simulink model "quadCorke"  (R2018a)
settings: Solver=VariableStepAuto  StartTime=0.0  StopTime=10.0  RelTol=1e-3
values from neighbouring files (symbols this model uses):
  MapMatrix = diag([ 1, -1, -1, -1, -1, 1, 1, -1, -1, -1, -1, 1])    [ScriptValues.m]
  x_d = 0    [ScriptValues.m]
  y_d = 0    [ScriptValues.m]
  z_d = 1    [ScriptValues.m]
undefined symbols (not defined in the file or in its folder): quadrotor
libraries: simulink x6, roblocks x2, aerolibutil x1
settings Model: Creator=dinies33  LastModifiedBy=giuseppe
settings ConfigComp: CovScope=ReferencedModels  CovIncludeTopModel=off

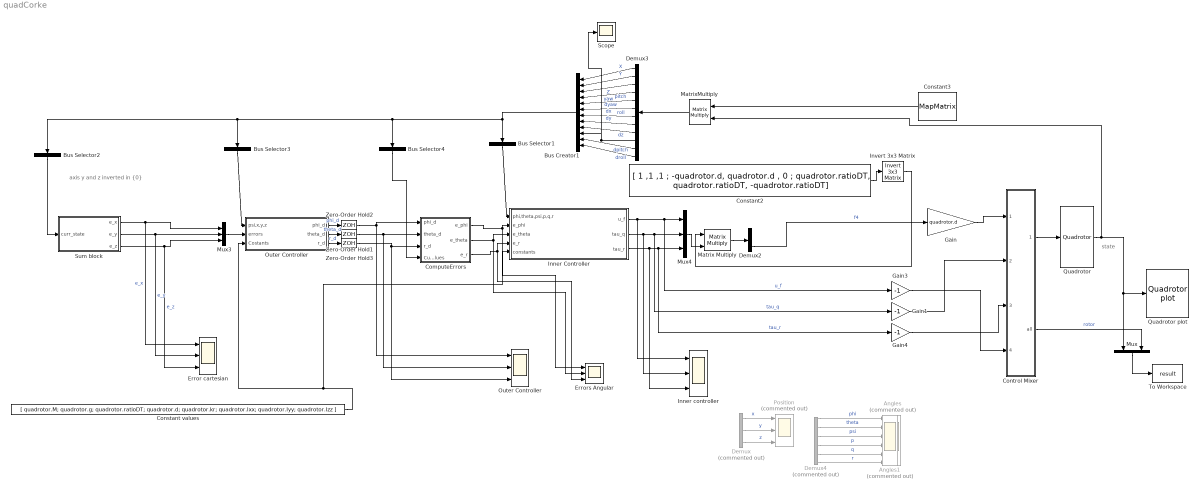
== system quadCorke ==
  note: axis y and z inverted in {0}
  note: state
  Angles : Scope  Commented=on  NumInputPorts=6
  Angles1 : Scope  Commented=on  NumInputPorts=6
  Bus Creator1 : BusCreator  Inputs='X','Y','Z','yaw','pitch','roll','dx','dy','dz','dyaw','dpitch','droll'
  Bus Selector1 : BusSelector  OutputSignals=roll,pitch,yaw,droll,dpitch,dyaw  OutputAsBus=on
  Bus Selector2 : BusSelector  OutputSignals=X,Y,Z  OutputAsBus=on
  Bus Selector3 : BusSelector  OutputSignals=yaw,X,Y,Z  OutputAsBus=on
  Bus Selector4 : BusSelector  OutputSignals=roll,pitch,dyaw  OutputAsBus=on
  "ComputeErrors " : Subsystem
  Constant values : Constant  Value=[ quadrotor.M; quadrotor.g; quadrotor.ratioDT; quadrotor.d; quadrotor.kr; quadrotor.Ixx; quadrotor.Iyy; quadrotor.Izz ]
  Constant2 : Constant  Value=[ 1 ,1 ,1 ; -quadrotor.d, quadrotor.d , 0 ; quadrotor.ratioDT, quadrotor.ratioDT, -quadrotor.ratioDT]
  Constant3 : Constant  Value=MapMatrix
  Control Mixer : Subsystem  AncestorBlock=roblocks/Vehicles/Control Mixer 4  mask{quad=quadrotor, maxrot=1000, minrot=5}
      mask prompts: quad "Quadrotor parameters"; maxrot "Maximum rotor speed (rad/s)"; minrot "Minimum rotor speed (rad/s)"
      mask help: Quadrotor control mixer
      mask Help:
      | Determine rotor speeds based on desired torques and thrust, and propellor model
      | 
      | <b>Inputs::</b>
      | tau<sub>x</sub> (1x1)    desired rolling torque [Nm]
      | 
      | tau<sub>y</sub> (1x1)    desired pitching torque [Nm]
      | tau<sub>z</sub> (1x1)    desired yawing torque [Nm]
      | T (1x1)          desired thrust [N]
      | 
      | <b>Outputs::</b>
      | 
      | w1 (1x1) angular velocity of rotor 1 [rad]
      | w2 (1x1) angular velocity of rotor 2 [rad]
      | w3 (1x1) angular velocity of rotor 3 [rad]
      | w4 (1x1) angular velocity of rotor 4 [rad]
      | 
      | <b>Notes::</b>
      | 
      | - Assumes the rotor labelling convention of RVC Fig 4.16.
      | - The quadrotor is underactuated and has only 4 inputs.
      mask Display:
      | port_label('output',1,'\varpi','texmode','on');
      | port_label('output',2,'\tau_a','texmode','on');
      | port_label('input',1,'\tau_x','texmode','on');
      | port_label('input',2,'\tau_y','texmode','on');
      | port_label('input',3,'\tau_z','texmode','on');
      | port_label('input',4,'T','texmode','on');
  Demux : Demux  Commented=on  Outputs=3
  Demux2 : Demux  Outputs=3
  Demux3 : Demux  Outputs=12
  Demux4 : Demux  Commented=on  Outputs=6
  Error cartesian : Scope  NumInputPorts=3
  Errors Angular : Scope  NumInputPorts=3
  Gain : Gain  Gain=quadrotor.d
  Gain1 : Gain  Gain=-1
  Gain3 : Gain  Gain=-1
  Gain4 : Gain  Gain=-1
  "Inner Controller " : Subsystem
  Inner controller : Scope  NumInputPorts=3
  Invert 3x3 Matrix : aerolibutil/Invert  3x3 Matrix
  Matrix Multiply : Product  Multiplication=Matrix(*)
  MatrixMultiply : Product  Multiplication=Matrix(*)
  Mux : Mux  Inputs=2
  Mux3 : Mux  Inputs=3
  Mux4 : Mux  Inputs=3
  Outer Controller : Scope  NumInputPorts=3
  "Outer Controller " : Subsystem
  Position : Scope  Commented=on  NumInputPorts=3
  Quadrotor : roblocks/Vehicles/Quadrotor  quad=quadrotor  x0=[0 0 -5]  groundflag=on
      link override Dynamics: FunctionName=corke_dynamics
  Quadrotor plot : roblocks/Vehicles/Quadrotor plot  quad=quadrotor  xydim=2  zdim=10
      link override Plotter: FunctionName=corke_plot  Parameters=[xydim, zdim], 1, 1,quad
  Scope : Scope
  Sum block : Subsystem
  To Workspace : ToWorkspace  VariableName=result  SampleTime=-1
  Zero-Order Hold1 : ZeroOrderHold  SampleTime=0.15
  Zero-Order Hold2 : ZeroOrderHold  SampleTime=0.15
  Zero-Order Hold3 : ZeroOrderHold  SampleTime=0.15
  wires:
  Control Mixer/2(all) -> Mux/2  "rotor"
  Mux/1 -> To Workspace/1
  Quadrotor/1 -> Quadrotor plot/1, Mux/1, MatrixMultiply/2
  Control Mixer/1(omega) -> Quadrotor/1
  Constant2/1 -> Invert 3x3 Matrix/1
  "Inner Controller "/1(u_f) -> Gain3/1, Mux4/1, Inner controller/1  "u_f"
  Demux4/6 -> Angles/6  "r"
  Demux4/1 -> Angles/1  "phi"
  Demux2/3 -> Gain/1  "f4"
  Sum block/1("e_x ") -> Error cartesian/1, Mux3/1  "e_x"
  Demux/2 -> Position/2  "y"
  Demux4/5 -> Angles/5  "q"
  "ComputeErrors "/1("e_phi ") -> Errors Angular/1, "Inner Controller "/2(e_phi)
  "ComputeErrors "/2(e_theta) -> Errors Angular/2, "Inner Controller "/3(e_theta)
  Matrix Multiply/1 -> Demux2/1
  Demux/1 -> Position/1  "x"
  "Inner Controller "/2(tau_q) -> Inner controller/2, Mux4/2, Gain1/1  "tau_q"
  Invert 3x3 Matrix/1 -> Matrix Multiply/1
  "Inner Controller "/3(tau_r) -> Inner controller/3, Gain4/1, Mux4/3  "tau_r"
  "Outer Controller "/3(r_d) -> Zero-Order Hold3/1  "r_d"
  "Outer Controller "/1("phi_d ") -> Zero-Order Hold2/1  "phi_d"
  "ComputeErrors "/3(e_r) -> Errors Angular/3, "Inner Controller "/4(e_r)
  Demux/3 -> Position/3  "z"
  Demux4/4 -> Angles/4  "p"
  Mux4/1 -> Matrix Multiply/2
  Demux4/3 -> Angles/3  "psi"
  Constant values/1 -> "Outer Controller "/3(Costants), "Inner Controller "/5(constants)
  Demux4/2 -> Angles/2  "theta"
  "Outer Controller "/2(theta_d) -> Zero-Order Hold1/1  "theta_d"
  Mux3/1 -> "Outer Controller "/2(errors)
  Sum block/2(e_y) -> Error cartesian/2, Mux3/2  "e_y"
  Sum block/3(e_z) -> Error cartesian/3, Mux3/3  "e_z"
  Gain/1 -> Control Mixer/1(tau roll)
  Bus Selector1/1 -> "Inner Controller "/1(phi,theta,psi,p,q,r)
  Bus Selector3/1 -> "Outer Controller "/1(psi,x,y,z)
  Bus Selector2/1 -> Sum block/1(curr_state)
  Bus Selector4/1 -> "ComputeErrors "/4(Curr_values)
  Constant3/1 -> MatrixMultiply/1
  Bus Creator1/1 -> Bus Selector2/1, Bus Selector3/1, Bus Selector4/1, Bus Selector1/1
  Demux3/3 -> Bus Creator1/3  "Z"
  Demux3/8 -> Bus Creator1/8  "dy"
  Demux3/7 -> Bus Creator1/7  "dx"
  Demux3/10 -> Scope/1, Bus Creator1/10  "dyaw"
  Demux3/5 -> Bus Creator1/5  "pitch"
  Demux3/2 -> Bus Creator1/2  "Y"
  Demux3/4 -> Bus Creator1/4  "yaw"
  Demux3/1 -> Bus Creator1/1  "X"
  Demux3/9 -> Bus Creator1/9  "dz"
  Demux3/11 -> Bus Creator1/11  "dpitch"
  Demux3/6 -> Bus Creator1/6  "roll"
  Demux3/12 -> Bus Creator1/12  "droll"
  MatrixMultiply/1 -> Demux3/1
  Gain1/1 -> Control Mixer/2(tau pitch)
  Gain3/1 -> Control Mixer/4(total thrust)
  Gain4/1 -> Control Mixer/3(tau yaw)
  Zero-Order Hold3/1 -> Outer Controller/3, "ComputeErrors "/3(r_d)
  Zero-Order Hold1/1 -> Outer Controller/2, "ComputeErrors "/2(theta_d)
  Zero-Order Hold2/1 -> "ComputeErrors "/1(phi_d), Outer Controller/1

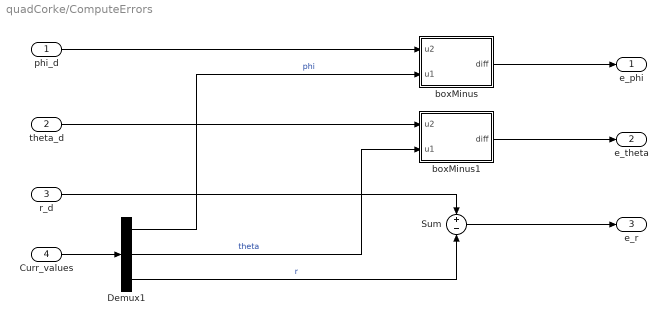
== system quadCorke/ComputeErrors  ==
  phi_d : Inport
  theta_d : Inport  Port=2
  r_d : Inport  Port=3
  Curr_values : Inport  Port=4
  Demux1 : Demux  Outputs=3
  Sum : Sum  Inputs=+-
  boxMinus : MATLAB Function  TreatAsAtomicUnit=on
  boxMinus1 : MATLAB Function  TreatAsAtomicUnit=on
  "e_phi " : Outport
  e_theta : Outport  Port=2
  e_r : Outport  Port=3
  wires:
  phi_d/1 -> boxMinus/1(u2)
  Demux1/1 -> boxMinus/2(u1)  "phi"
  theta_d/1 -> boxMinus1/1(u2)
  Demux1/2 -> boxMinus1/2(u1)  "theta"
  r_d/1 -> Sum/1
  Demux1/3 -> Sum/2  "r"
  Sum/1 -> e_r/1
  boxMinus1/1(diff) -> e_theta/1
  boxMinus/1(diff) -> "e_phi "/1
  Curr_values/1 -> Demux1/1

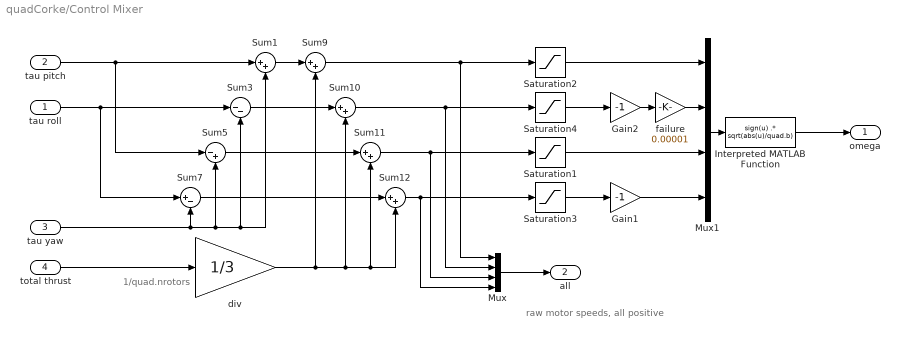
== system quadCorke/Control Mixer ==
  note: 1/quad.nrotors
  note: raw motor speeds, all positive
  tau roll : Inport
  tau pitch : Inport  Port=2
  tau yaw : Inport  Port=3
  total thrust : Inport  Port=4
  Gain1 : Gain  Gain=-1
  Gain2 : Gain  Gain=-1
  Interpreted MATLAB Function : MATLABFcn  MATLABFcn=sign(u) .* sqrt(abs(u)/quad.b)
  Mux : Mux
  Mux1 : Mux
  Saturation{1..4} (4 alike) : Saturate  UpperLimit=maxrot  LowerLimit=minrot
  Sum{1,9..12} (5 alike) : Sum  Inputs=|++  SaturateOnIntegerOverflow=on  InputSameDT=on  OutDataTypeStr=Inherit: Same as first input
  Sum3 : Sum  Inputs=|--  SaturateOnIntegerOverflow=on  InputSameDT=on  OutDataTypeStr=Inherit: Same as first input
  Sum5 : Sum  Inputs=|-+  SaturateOnIntegerOverflow=on  InputSameDT=on  OutDataTypeStr=Inherit: Same as first input
  Sum7 : Sum  Inputs=|+-  SaturateOnIntegerOverflow=on  InputSameDT=on  OutDataTypeStr=Inherit: Same as first input
  div : Gain  Gain=1/3
  failure : Gain  Gain=0.00001
  omega : Outport
  all : Outport  Port=2
  wires:
  div/1 -> Sum11/2, Sum12/2, Sum10/2, Sum9/2
  Interpreted MATLAB Function/1 -> omega/1
  Mux1/1 -> Interpreted MATLAB Function/1
  tau yaw/1 -> Sum7/2, Sum5/2, Sum3/2, Sum1/2
  Saturation2/1 -> Mux1/1
  Saturation4/1 -> Gain2/1
  Saturation1/1 -> Mux1/3
  Saturation3/1 -> Gain1/1
  tau pitch/1 -> Sum1/1, Sum5/1
  Sum1/1 -> Sum9/1
  Sum3/1 -> Sum10/1
  Sum5/1 -> Sum11/1
  Sum7/1 -> Sum12/1
  Sum9/1 -> Saturation2/1, Mux/1
  Sum10/1 -> Mux/2, Saturation4/1
  Sum11/1 -> Mux/3, Saturation1/1
  Sum12/1 -> Mux/4, Saturation3/1
  total thrust/1 -> div/1
  tau roll/1 -> Sum3/1, Sum7/1
  Mux/1 -> all/1
  Gain1/1 -> Mux1/4
  Gain2/1 -> failure/1
  failure/1 -> Mux1/2

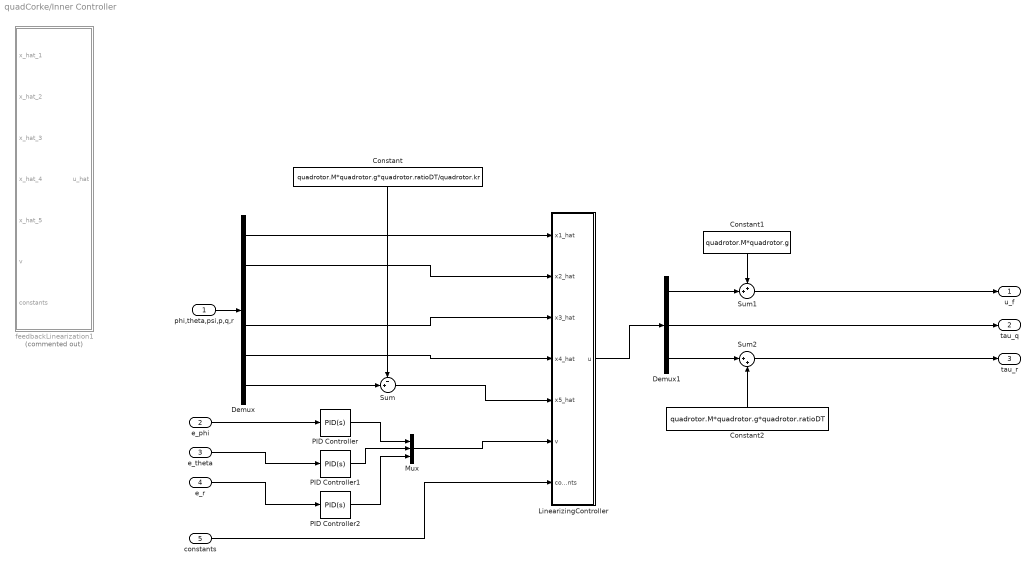
== system quadCorke/Inner Controller  ==
  phi,theta,psi,p,q,r : Inport
  e_phi : Inport  Port=2
  e_theta : Inport  Port=3
  e_r : Inport  Port=4
  constants : Inport  Port=5
  Constant : Constant  Value=quadrotor.M*quadrotor.g*quadrotor.ratioDT/quadrotor.kr
  Constant1 : Constant  Value=quadrotor.M*quadrotor.g
  Constant2 : Constant  Value=quadrotor.M*quadrotor.g*quadrotor.ratioDT
  Demux : Demux  Outputs=6
  Demux1 : Demux  Outputs=3
  LinearizingController : MATLAB Function  TreatAsAtomicUnit=on
  Mux : Mux  Inputs=3
  PID Controller : simulink/Continuous/PID Controller  Controller=PID  TimeDomain=Continuous-time  SampleTime=-1  IntegratorMethod=Forward Euler  FilterMethod=Forward Euler  Form=Parallel  UseFilter=on  ControllerParametersSource=internal  P=1  I=1  D=0  N=100  InitialConditionSource=internal  InitialConditionForIntegrator=0  InitialConditionForFilter=0  ExternalReset=none  LimitOutput=off  UpperSaturationLimit=inf  LowerSaturationLimit=-inf  LinearizeAsGain=on  AntiWindupMode=none  Kb=1  TrackingMode=off  Kt=1  PParamMin=[]  PParamMax=[]  IParamMin=[]  IParamMax=[]  DParamMin=[]  DParamMax=[]  NParamMin=[]  NParamMax=[]  KbParamMin=[]  KbParamMax=[]  KtParamMin=[]  KtParamMax=[]  POutMin=[]  POutMax=[]  IOutMin=[]  IOutMax=[]  DOutMin=[]  DOutMax=[]  NOutMin=[]  NOutMax=[]  KbOutMin=[]  KbOutMax=[]  KtOutMin=[]  KtOutMax=[]  IntegratorOutMin=[]  IntegratorOutMax=[]  FilterOutMin=[]  FilterOutMax=[]  SumOutMin=[]  SumOutMax=[]  SumI1OutMin=[]  SumI1OutMax=[]  SumI2OutMin=[]  SumI2OutMax=[]  SumI3OutMin=[]  SumI3OutMax=[]  SumDOutMin=[]  SumDOutMax=[]  SaturationOutMin=[]  SaturationOutMax=[]  IntegratorContinuousStateAttributes=''  IntegratorStateMustResolveToSignalObject=off  IntegratorRTWStateStorageClass=Auto  FilterContinuousStateAttributes=''  FilterStateMustResolveToSignalObject=off  FilterRTWStateStorageClass=Auto  DifferentiatorICPrevScaledInput=0  DifferentiatorOutMin=[]  DifferentiatorOutMax=[]  FilterDiffOutCoefMin=[]  FilterDiffOutCoefMax=[]  SumDenOutMin=[]  SumDenOutMax=[]  SumNumOutMin=[]  SumNumOutMax=[]  ReciprocalOutMin=[]  ReciprocalOutMax=[]  DivideOutMin=[]  DivideOutMax=[]  TunerSelectOption=Transfer Function Based (PID Tuner App)
  PID Controller1 : simulink/Continuous/PID Controller  Controller=PID  TimeDomain=Continuous-time  SampleTime=-1  IntegratorMethod=Forward Euler  FilterMethod=Forward Euler  Form=Parallel  UseFilter=on  ControllerParametersSource=internal  P=1  I=1  D=0  N=100  InitialConditionSource=internal  InitialConditionForIntegrator=0  InitialConditionForFilter=0  ExternalReset=none  LimitOutput=off  UpperSaturationLimit=inf  LowerSaturationLimit=-inf  LinearizeAsGain=on  AntiWindupMode=none  Kb=1  TrackingMode=off  Kt=1  PParamMin=[]  PParamMax=[]  IParamMin=[]  IParamMax=[]  DParamMin=[]  DParamMax=[]  NParamMin=[]  NParamMax=[]  KbParamMin=[]  KbParamMax=[]  KtParamMin=[]  KtParamMax=[]  POutMin=[]  POutMax=[]  IOutMin=[]  IOutMax=[]  DOutMin=[]  DOutMax=[]  NOutMin=[]  NOutMax=[]  KbOutMin=[]  KbOutMax=[]  KtOutMin=[]  KtOutMax=[]  IntegratorOutMin=[]  IntegratorOutMax=[]  FilterOutMin=[]  FilterOutMax=[]  SumOutMin=[]  SumOutMax=[]  SumI1OutMin=[]  SumI1OutMax=[]  SumI2OutMin=[]  SumI2OutMax=[]  SumI3OutMin=[]  SumI3OutMax=[]  SumDOutMin=[]  SumDOutMax=[]  SaturationOutMin=[]  SaturationOutMax=[]  IntegratorContinuousStateAttributes=''  IntegratorStateMustResolveToSignalObject=off  IntegratorRTWStateStorageClass=Auto  FilterContinuousStateAttributes=''  FilterStateMustResolveToSignalObject=off  FilterRTWStateStorageClass=Auto  DifferentiatorICPrevScaledInput=0  DifferentiatorOutMin=[]  DifferentiatorOutMax=[]  FilterDiffOutCoefMin=[]  FilterDiffOutCoefMax=[]  SumDenOutMin=[]  SumDenOutMax=[]  SumNumOutMin=[]  SumNumOutMax=[]  ReciprocalOutMin=[]  ReciprocalOutMax=[]  DivideOutMin=[]  DivideOutMax=[]  TunerSelectOption=Transfer Function Based (PID Tuner App)
  PID Controller2 : simulink/Continuous/PID Controller  Controller=PID  TimeDomain=Continuous-time  SampleTime=-1  IntegratorMethod=Forward Euler  FilterMethod=Forward Euler  Form=Parallel  UseFilter=on  ControllerParametersSource=internal  P=1  I=1  D=0  N=100  InitialConditionSource=internal  InitialConditionForIntegrator=0  InitialConditionForFilter=0  ExternalReset=none  LimitOutput=off  UpperSaturationLimit=inf  LowerSaturationLimit=-inf  LinearizeAsGain=on  AntiWindupMode=none  Kb=1  TrackingMode=off  Kt=1  PParamMin=[]  PParamMax=[]  IParamMin=[]  IParamMax=[]  DParamMin=[]  DParamMax=[]  NParamMin=[]  NParamMax=[]  KbParamMin=[]  KbParamMax=[]  KtParamMin=[]  KtParamMax=[]  POutMin=[]  POutMax=[]  IOutMin=[]  IOutMax=[]  DOutMin=[]  DOutMax=[]  NOutMin=[]  NOutMax=[]  KbOutMin=[]  KbOutMax=[]  KtOutMin=[]  KtOutMax=[]  IntegratorOutMin=[]  IntegratorOutMax=[]  FilterOutMin=[]  FilterOutMax=[]  SumOutMin=[]  SumOutMax=[]  SumI1OutMin=[]  SumI1OutMax=[]  SumI2OutMin=[]  SumI2OutMax=[]  SumI3OutMin=[]  SumI3OutMax=[]  SumDOutMin=[]  SumDOutMax=[]  SaturationOutMin=[]  SaturationOutMax=[]  IntegratorContinuousStateAttributes=''  IntegratorStateMustResolveToSignalObject=off  IntegratorRTWStateStorageClass=Auto  FilterContinuousStateAttributes=''  FilterStateMustResolveToSignalObject=off  FilterRTWStateStorageClass=Auto  DifferentiatorICPrevScaledInput=0  DifferentiatorOutMin=[]  DifferentiatorOutMax=[]  FilterDiffOutCoefMin=[]  FilterDiffOutCoefMax=[]  SumDenOutMin=[]  SumDenOutMax=[]  SumNumOutMin=[]  SumNumOutMax=[]  ReciprocalOutMin=[]  ReciprocalOutMax=[]  DivideOutMin=[]  DivideOutMax=[]  TunerSelectOption=Transfer Function Based (PID Tuner App)
  Sum : Sum  Inputs=-+|
  Sum1 : Sum  Inputs=++|
  Sum2 : Sum  Inputs=|++
  feedbackLinearization1 : MATLAB Function  Commented=on  TreatAsAtomicUnit=on
  u_f : Outport
  tau_q : Outport  Port=2
  tau_r : Outport  Port=3
  wires:
  phi,theta,psi,p,q,r/1 -> Demux/1
  Demux/1 -> LinearizingController/1(x1_hat)
  Demux/2 -> LinearizingController/2(x2_hat)
  Demux/4 -> LinearizingController/3(x3_hat)
  Demux/5 -> LinearizingController/4(x4_hat)
  Constant/1 -> Sum/1
  Sum/1 -> LinearizingController/5(x5_hat)
  Demux1/3 -> Sum2/1
  Demux1/1 -> Sum1/2
  Constant1/1 -> Sum1/1
  Sum1/1 -> u_f/1
  Demux1/2 -> tau_q/1
  Constant2/1 -> Sum2/2
  Sum2/1 -> tau_r/1
  constants/1 -> LinearizingController/7(constants)
  Demux/6 -> Sum/2
  e_theta/1 -> PID Controller1/1
  PID Controller2/1 -> Mux/3
  PID Controller/1 -> Mux/1
  Mux/1 -> LinearizingController/6(v)
  PID Controller1/1 -> Mux/2
  e_r/1 -> PID Controller2/1
  e_phi/1 -> PID Controller/1
  LinearizingController/1(u) -> Demux1/1

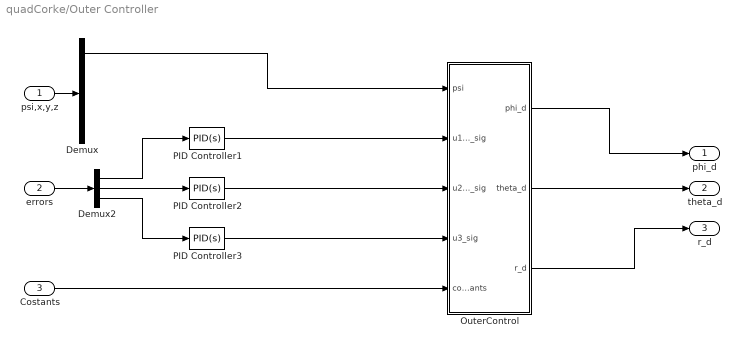
== system quadCorke/Outer Controller  ==
  psi,x,y,z : Inport  SampleTime=0.1
  errors : Inport  Port=2
  Costants : Inport  Port=3
  Demux : Demux
  Demux2 : Demux  Outputs=3
  OuterControl : MATLAB Function  TreatAsAtomicUnit=on
  PID Controller1 : simulink/Continuous/PID Controller  Controller=PID  TimeDomain=Continuous-time  SampleTime=-1  IntegratorMethod=Forward Euler  FilterMethod=Forward Euler  Form=Parallel  UseFilter=on  ControllerParametersSource=internal  P=0.939601981976548  I=0.0298455660718895  D=4.45438528962657  N=508.848592355901  InitialConditionSource=internal  InitialConditionForIntegrator=0  InitialConditionForFilter=0  ExternalReset=none  LimitOutput=off  UpperSaturationLimit=inf  LowerSaturationLimit=-inf  LinearizeAsGain=on  AntiWindupMode=none  Kb=1  TrackingMode=off  Kt=1  PParamMin=[]  PParamMax=[]  IParamMin=[]  IParamMax=[]  DParamMin=[]  DParamMax=[]  NParamMin=[]  NParamMax=[]  KbParamMin=[]  KbParamMax=[]  KtParamMin=[]  KtParamMax=[]  POutMin=[]  POutMax=[]  IOutMin=[]  IOutMax=[]  DOutMin=[]  DOutMax=[]  NOutMin=[]  NOutMax=[]  KbOutMin=[]  KbOutMax=[]  KtOutMin=[]  KtOutMax=[]  IntegratorOutMin=[]  IntegratorOutMax=[]  FilterOutMin=[]  FilterOutMax=[]  SumOutMin=[]  SumOutMax=[]  SumI1OutMin=[]  SumI1OutMax=[]  SumI2OutMin=[]  SumI2OutMax=[]  SumI3OutMin=[]  SumI3OutMax=[]  SumDOutMin=[]  SumDOutMax=[]  SaturationOutMin=[]  SaturationOutMax=[]  IntegratorContinuousStateAttributes=''  IntegratorStateMustResolveToSignalObject=off  IntegratorRTWStateStorageClass=Auto  FilterContinuousStateAttributes=''  FilterStateMustResolveToSignalObject=off  FilterRTWStateStorageClass=Auto  DifferentiatorICPrevScaledInput=0  DifferentiatorOutMin=[]  DifferentiatorOutMax=[]  FilterDiffOutCoefMin=[]  FilterDiffOutCoefMax=[]  SumDenOutMin=[]  SumDenOutMax=[]  SumNumOutMin=[]  SumNumOutMax=[]  ReciprocalOutMin=[]  ReciprocalOutMax=[]  DivideOutMin=[]  DivideOutMax=[]  TunerSelectOption=Transfer Function Based (PID Tuner App)
  PID Controller2 : simulink/Continuous/PID Controller  Controller=PID  TimeDomain=Continuous-time  SampleTime=-1  IntegratorMethod=Forward Euler  FilterMethod=Forward Euler  Form=Parallel  UseFilter=on  ControllerParametersSource=internal  P=0.942155734377191  I=0.0299673249963071  D=4.46043448837536  N=509.539625142761  InitialConditionSource=internal  InitialConditionForIntegrator=0  InitialConditionForFilter=0  ExternalReset=none  LimitOutput=off  UpperSaturationLimit=inf  LowerSaturationLimit=-inf  LinearizeAsGain=on  AntiWindupMode=none  Kb=1  TrackingMode=off  Kt=1  PParamMin=[]  PParamMax=[]  IParamMin=[]  IParamMax=[]  DParamMin=[]  DParamMax=[]  NParamMin=[]  NParamMax=[]  KbParamMin=[]  KbParamMax=[]  KtParamMin=[]  KtParamMax=[]  POutMin=[]  POutMax=[]  IOutMin=[]  IOutMax=[]  DOutMin=[]  DOutMax=[]  NOutMin=[]  NOutMax=[]  KbOutMin=[]  KbOutMax=[]  KtOutMin=[]  KtOutMax=[]  IntegratorOutMin=[]  IntegratorOutMax=[]  FilterOutMin=[]  FilterOutMax=[]  SumOutMin=[]  SumOutMax=[]  SumI1OutMin=[]  SumI1OutMax=[]  SumI2OutMin=[]  SumI2OutMax=[]  SumI3OutMin=[]  SumI3OutMax=[]  SumDOutMin=[]  SumDOutMax=[]  SaturationOutMin=[]  SaturationOutMax=[]  IntegratorContinuousStateAttributes=''  IntegratorStateMustResolveToSignalObject=off  IntegratorRTWStateStorageClass=Auto  FilterContinuousStateAttributes=''  FilterStateMustResolveToSignalObject=off  FilterRTWStateStorageClass=Auto  DifferentiatorICPrevScaledInput=0  DifferentiatorOutMin=[]  DifferentiatorOutMax=[]  FilterDiffOutCoefMin=[]  FilterDiffOutCoefMax=[]  SumDenOutMin=[]  SumDenOutMax=[]  SumNumOutMin=[]  SumNumOutMax=[]  ReciprocalOutMin=[]  ReciprocalOutMax=[]  DivideOutMin=[]  DivideOutMax=[]  TunerSelectOption=Transfer Function Based (PID Tuner App)
  PID Controller3 : simulink/Continuous/PID Controller  Controller=PID  TimeDomain=Continuous-time  SampleTime=-1  IntegratorMethod=Forward Euler  FilterMethod=Forward Euler  Form=Parallel  UseFilter=on  ControllerParametersSource=internal  P=0.939353785780563  I=0.0298337412778135  D=4.45379693701357  N=508.781381652965  InitialConditionSource=internal  InitialConditionForIntegrator=0  InitialConditionForFilter=0  ExternalReset=none  LimitOutput=off  UpperSaturationLimit=inf  LowerSaturationLimit=-inf  LinearizeAsGain=on  AntiWindupMode=none  Kb=1  TrackingMode=off  Kt=1  PParamMin=[]  PParamMax=[]  IParamMin=[]  IParamMax=[]  DParamMin=[]  DParamMax=[]  NParamMin=[]  NParamMax=[]  KbParamMin=[]  KbParamMax=[]  KtParamMin=[]  KtParamMax=[]  POutMin=[]  POutMax=[]  IOutMin=[]  IOutMax=[]  DOutMin=[]  DOutMax=[]  NOutMin=[]  NOutMax=[]  KbOutMin=[]  KbOutMax=[]  KtOutMin=[]  KtOutMax=[]  IntegratorOutMin=[]  IntegratorOutMax=[]  FilterOutMin=[]  FilterOutMax=[]  SumOutMin=[]  SumOutMax=[]  SumI1OutMin=[]  SumI1OutMax=[]  SumI2OutMin=[]  SumI2OutMax=[]  SumI3OutMin=[]  SumI3OutMax=[]  SumDOutMin=[]  SumDOutMax=[]  SaturationOutMin=[]  SaturationOutMax=[]  IntegratorContinuousStateAttributes=''  IntegratorStateMustResolveToSignalObject=off  IntegratorRTWStateStorageClass=Auto  FilterContinuousStateAttributes=''  FilterStateMustResolveToSignalObject=off  FilterRTWStateStorageClass=Auto  DifferentiatorICPrevScaledInput=0  DifferentiatorOutMin=[]  DifferentiatorOutMax=[]  FilterDiffOutCoefMin=[]  FilterDiffOutCoefMax=[]  SumDenOutMin=[]  SumDenOutMax=[]  SumNumOutMin=[]  SumNumOutMax=[]  ReciprocalOutMin=[]  ReciprocalOutMax=[]  DivideOutMin=[]  DivideOutMax=[]  TunerSelectOption=Transfer Function Based (PID Tuner App)
  "phi_d " : Outport
  theta_d : Outport  Port=2
  r_d : Outport  Port=3
  wires:
  psi,x,y,z/1 -> Demux/1
  Demux/1 -> OuterControl/1(psi)
  OuterControl/3(r_d) -> r_d/1
  OuterControl/1(phi_d) -> "phi_d "/1
  OuterControl/2(theta_d) -> theta_d/1
  Costants/1 -> OuterControl/5(constants)
  PID Controller3/1 -> OuterControl/4(u3_sig)
  PID Controller2/1 -> OuterControl/3(u2_sig_sig)
  PID Controller1/1 -> OuterControl/2(u1_sig_sig)
  errors/1 -> Demux2/1
  Demux2/1 -> PID Controller1/1
  Demux2/2 -> PID Controller2/1
  Demux2/3 -> PID Controller3/1

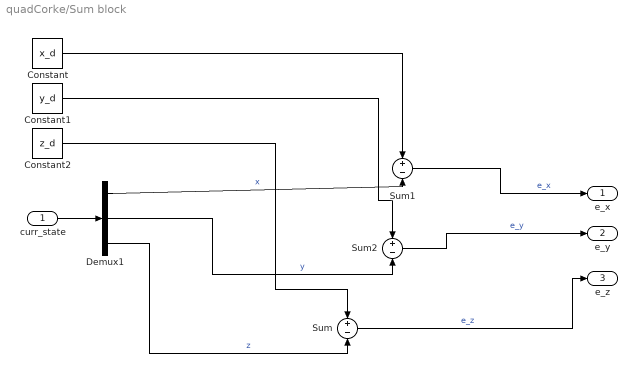
== system quadCorke/Sum block ==
  curr_state : Inport
  Constant : Constant  Value=x_d
  Constant1 : Constant  Value=y_d
  Constant2 : Constant  Value=z_d
  Demux1 : Demux  Outputs=3
  Sum : Sum  Inputs=+-
  Sum1 : Sum  Inputs=+-
  Sum2 : Sum  Inputs=+-
  "e_x " : Outport
  e_y : Outport  Port=2
  e_z : Outport  Port=3
  wires:
  Demux1/3 -> Sum/2  "z"
  curr_state/1 -> Demux1/1
  Constant2/1 -> Sum/1
  Constant1/1 -> Sum2/1
  Constant/1 -> Sum1/1
  Demux1/2 -> Sum2/2  "y"
  Demux1/1 -> Sum1/2  "x"
  Sum/1 -> e_z/1  "e_z"
  Sum2/1 -> e_y/1  "e_y"
  Sum1/1 -> "e_x "/1  "e_x"

== matlab function quadCorke/Inner Controller /LinearizingController ==
  data: x1_hat input; u output; x2_hat input; x3_hat input; x4_hat input; x5_hat input; v input; constants input
function u = fcn(x1_hat,x2_hat,x3_hat,x4_hat,x5_hat,v, constants)

m= constants(1,1);
g= constants(2,1);
d= constants(3,1);
l= constants(4,1);
kr= constants(5,1);
Ixx= constants(6,1);
Iyy= constants(7,1);
Izz= constants(8,1);

alfa = zeros(3,1);

alfa(1,1) = (2*Ixx*((kr*x3_hat - x4_hat*(x5_hat + (d*g*m)/kr)*(Ixx - Izz))/Ixx + (sin(x1_hat)*tan(x2_hat)*(x5_hat + (d*g*m)/kr) - x4_hat*cos(x1_hat)*tan(x2_hat))*(x3_hat + cos(x1_hat)*tan(x2_hat)*(x5_hat + (d*g*m)/kr) + x4_hat*sin(x1_hat)*tan(x2_hat)) + (sin(x1_hat)*(x5_hat + (d*g*m)/kr) - x4_hat*cos(x1_hat))*(cos(x1_hat)*(x5_hat + (d*g*m)/kr)*(tan(x2_hat)^2 + 1) + x4_hat*sin(x1_hat)*(tan(x2_hat)^2 + 1)) + (sin(x1_hat)*tan(x2_hat)*(kr*x4_hat + x3_hat*(x5_hat + (d*g*m)/kr)*(Ixx - Izz)))/Ixx + (kr*x5_hat*cos(x1_hat)*tan(x2_hat))/Izz))/l - (2*Ixx*sin(x1_hat)*tan(x2_hat)*((cos(x1_hat)*(x5_hat + (d*g*m)/kr) + x4_hat*sin(x1_hat))*(x3_hat + cos(x1_hat)*tan(x2_hat)*(x5_hat + (d*g*m)/kr) + x4_hat*sin(x1_hat)*tan(x2_hat)) + (cos(x1_hat)*(kr*x4_hat + x3_hat*(x5_hat + (d*g*m)/kr)*(Ixx - Izz)))/Ixx - (kr*x5_hat*sin(x1_hat))/Izz))/(l*cos(x1_hat)) - (kr*x5_hat*(2*Ixx*d*cos(x1_hat)^2*tan(x2_hat) - Izz*l*cos(x1_hat) + 2*Ixx*d*sin(x1_hat)^2*tan(x2_hat)))/(Izz*d*l*cos(x1_hat));
alfa(2,1) = (Ixx*((cos(x1_hat)*(x5_hat + (d*g*m)/kr) + x4_hat*sin(x1_hat))*(x3_hat + cos(x1_hat)*tan(x2_hat)*(x5_hat + (d*g*m)/kr) + x4_hat*sin(x1_hat)*tan(x2_hat)) + (cos(x1_hat)*(kr*x4_hat + x3_hat*(x5_hat + (d*g*m)/kr)*(Ixx - Izz)))/Ixx - (kr*x5_hat*sin(x1_hat))/Izz))/cos(x1_hat) + (Ixx*kr*x5_hat*sin(x1_hat))/(Izz*cos(x1_hat));
alfa(3,1) = kr*x5_hat;

beta =  [
         (2*Ixx)/l, -(2*Ixx*sin(x1_hat)*sin(x2_hat))/(l*cos(x1_hat)*cos(x2_hat)), -(2*Ixx*d*sin(x2_hat)-Izz*l*cos(x1_hat)*cos(x2_hat))/(d*l*cos(x1_hat)*cos(x2_hat));
         0,                                              Ixx/cos(x1_hat),                                                        (Ixx*sin(x1_hat))/cos(x1_hat);
         0,                                                            0,                                                                                  Izz];

u = alfa + beta*v;

== matlab function quadCorke/Inner Controller /feedbackLinearization1 ==
  data: x_hat_1 input; x_hat_2 input; x_hat_3 input; x_hat_4 input; x_hat_5 input; u_hat output; v input; constants input
function u_hat= fcn(x_hat_1,x_hat_2,x_hat_3,x_hat_4,x_hat_5, v, constants)

m= constants(1,1);
g= constants(2,1);
d= constants(3,1);
l= constants(4,1);
kr= constants(5,1);
Ixx= constants(6,1);
Iyy= constants(7,1);
Izz= constants(8,1);

x1 = x_hat_1;
x2 = x_hat_2;
x3 = x_hat_3;
x4 = x_hat_4;
x5 = x_hat_5;

alfa = zeros(3,1);

alfa(1,1) = -2*l*Izz*kr^2*(Ixx*(-1/4*cos(x2)^-2*Izz*(2*d^2*g^2*m^2*...
    (sin(2*x1) + x1 + cos(2*x2)*(-4*sin(x1) +x1 ) -sin(2*x2)*x2*tan(x1))+...
    2*d*g*m*kr*( -3*x4 - 4*cos(2*x2)*sin(x1)*x5+ cos(x1)^-1 *(2*x4- ...
    cos(3*x1)*x4 + 2*cos(2*x1)*cos(2*x2)*x4 + sin(3*x1)*x5)+ ...
    (2*sin(2*x2)*x3+ x5)* tan(x1))+ kr^2*( -6*x4*x5 - cos(x1)^-1 *...
    (2 *sin(2*x2)*x3*x4 + 2*cos(3*x1)*x4*x5 + sin(3*x1)*(x4- x5)*(x4+x5))+...
    (x5^2 - 3*x4^2+2*cos(2*x2)*x4^2)*tan(x1))) - cos(x1)^-1*kr^3*x5*tan(x2))+...
    Izz*( kr^2*( cos(x1)^-1 *kr*x5*tan(x2) - d*g*m*( x2+ cos(x1)^-1 *(-1+...
    sin(x1)*x1)*tan(x2)))+Izz*( -kr^2 *x4*x5+d*g*m*kr*(-x4+cos(x1)*x4-...
    sin(x1)*x5+x3*tan(x1)*tan(x2)+ sin(x1)*( x5+ x4*tan(x1))*tan(x2)^2)+...
    d^2 * g^2 * m^2 * (x1- x2*tan(x1)*tan(x2)+ sin(x1)* (-1+ tan(x2)^2)))));

alfa(2,1) =  Izz*kr^2*(Ixx*(-kr^3* x5*tan(x1)+ Izz*( d^2*g^2*m^2*(cos(x1)^-1* ...
    x2 + (-2+cos(x1)) *tan(x2)) + kr^2*(x3*(2*x5+x4*tan(x1))+ cos(x1)^-1*(sin(x1)*...
    x4+ cos(x1)*x5)^2 * tan(x2)) + 2*d*g*m*kr*( x3 - cos(x1)^-1*x3+ (sin(x1)*x4- ...
    x5 +cos(x1)*x5 - x4*tan(x1))* tan(x2)))) + Izz * ( cos(x1)^-1 * kr^2*...
    (d*g*m*( sin(x1) - x1) + sin(x1)*kr*x5) + Izz *(-kr^2*x3*x5+ d^2*g^2*m^2*...
    (-cos(x1)^-1*x2 + tan(x2))+ d*g*m*kr*((-1+ cos(x1)^-1)*x3+(x5+x4*tan(x1))*...
    tan(x2)))));

alfa(3,1) = 0;

% elem 2,2 is dubious, on the paper is written as SCx1, what is S ?
beta = [
    1 , -2*(tan(x1)*tan(x2))/l , -2*(cos(x1)^-1*Ixx*tan(x2))/(l*Izz) ; 
    0 ,  1/cos(x1) , Ixx*tan(x1)/Izz ;
    0 ,  0  ,   1;
    ];


u_hat = alfa + beta* v;

== matlab function quadCorke/ComputeErrors /boxMinus ==
  data: u2 input; diff output; u1 input
function diff = fcn(u2, u1)

R2 = [cos(u2) -sin(u2);
      sin(u2) cos(u2)];

R1 = [cos(-u1) -sin(-u1);
      sin(-u1) cos(-u1)];

R = R2*R1;

diff = atan2(R(2,1), R(1,1));

== matlab function quadCorke/ComputeErrors /boxMinus1 ==
  data: u2 input; diff output; u1 input
function diff = fcn(u2, u1)

R2 = [cos(u2) -sin(u2);
      sin(u2) cos(u2)];

R1 = [cos(-u1) -sin(-u1);
      sin(-u1) cos(-u1)];

R = R2*R1;

diff = atan2(R(2,1), R(1,1));

== matlab function quadCorke/Outer Controller /OuterControl ==
  data: psi input; phi_d output; u1_sig_sig input; u2_sig_sig input; u3_sig input; theta_d output; r_d output; constants input
function [phi_d , theta_d , r_d ] = fcn(psi, u1_sig_sig, u2_sig_sig, u3_sig, constants)

m= constants(1,1);
d= constants(3,1);
kr= constants(5,1);

R = [sin(psi), -cos(psi);
    cos(psi), sin(psi)];


u12 = R*[u1_sig_sig;u2_sig_sig];


r_d = u3_sig*d*m/kr;
phi_d_raw= u12(1,1)/u3_sig;
theta_d_raw = u12(2,1)/u3_sig;

phi_d = mod( phi_d_raw, 2*pi);
theta_d = mod( theta_d_raw, 2*pi);
